simulink model "Engine"  (R2018a)
settings: Solver=VariableStepAuto  StartTime=0.0  StopTime=0  RelTol=1e-3
settings Model: Creator=josefl  LastModifiedBy=josefl

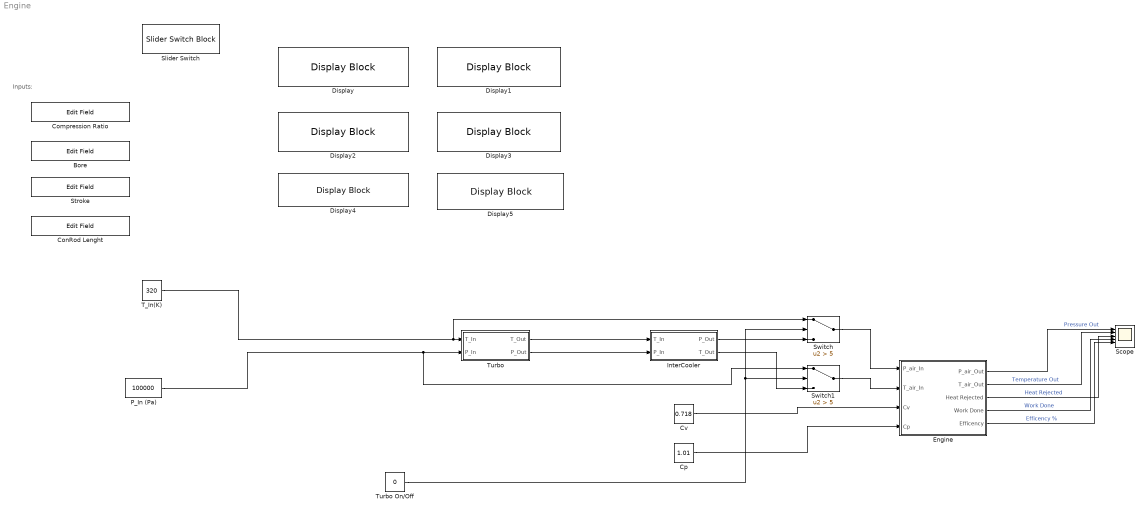
== system Engine ==
  note: Inputs:
  Bore : EditField  WebBlockId=61  LabelPosition=Hide  Alignment=Center
  "Compression Ratio " : EditField  WebBlockId=60  LabelPosition=Hide  Alignment=Center
  ConRod Lenght : EditField  WebBlockId=93  LabelPosition=Hide  Alignment=Center
  "Cp " : Constant  Value=1.01
  Cv : Constant  Value=0.718
  Display : DisplayBlock  WebBlockId=84
  Display1 : DisplayBlock  WebBlockId=85
  Display2 : DisplayBlock  WebBlockId=86
  Display3 : DisplayBlock  WebBlockId=87
  Display4 : DisplayBlock  WebBlockId=88
  Display5 : DisplayBlock  WebBlockId=89  LabelPosition=Hide
  "Engine " : Subsystem
  InterCooler : Subsystem
  "P_In (Pa) " : Constant  Value=100000
  Scope : Scope  NumInputPorts=5
  Slider Switch : SliderSwitchBlock  WebBlockId=64
      settings: Values={{'Off', 'On'}, [0 6]}
  "Stroke " : EditField  WebBlockId=62  LabelPosition=Hide  Alignment=Center
  Switch : Switch  Criteria=u2 > Threshold  Threshold=5
  Switch1 : Switch  Criteria=u2 > Threshold  Threshold=5
  "T_In(K) " : Constant  Value=320
  "Turbo " : Subsystem
  "Turbo On/Off " : Constant  Value=0
  wires:
  "Engine "/1("P_air_Out ") -> Scope/1  "Pressure Out"
  "Engine "/2("T_air_Out ") -> Scope/2  "Temperature Out"
  Cv/1 -> "Engine "/3(Cv)
  "Cp "/1 -> "Engine "/4("Cp ")
  "Engine "/3("Heat Rejected ") -> Scope/3  "Heat Rejected"
  "Engine "/4(Work Done) -> Scope/4  "Work Done"
  "Engine "/5(Efficency) -> Scope/5  "Efficency %"
  "P_In (Pa) "/1 -> Switch1/1, "Turbo "/2(P_In)
  "T_In(K) "/1 -> Switch/1, "Turbo "/1(T_In)
  "Turbo "/1(T_Out) -> InterCooler/1(T_In)
  "Turbo "/2(P_Out) -> InterCooler/2(P_In)
  InterCooler/1(P_Out) -> Switch/3
  Switch1/1 -> "Engine "/2("T_air_In ")
  Switch/1 -> "Engine "/1("P_air_In ")
  "Turbo On/Off "/1 -> Switch/2, Switch1/2
  InterCooler/2(T_Out) -> Switch1/3

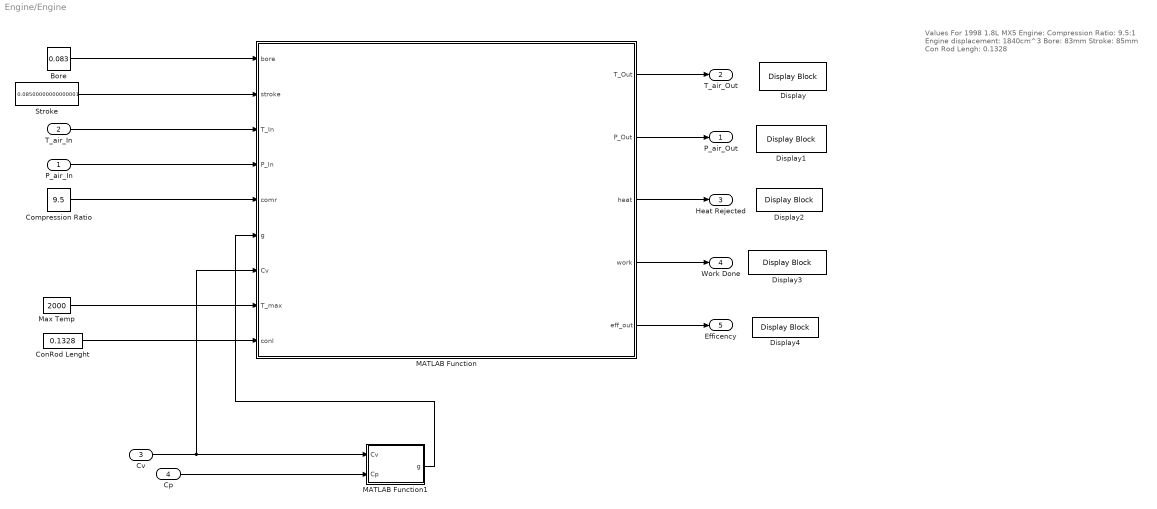
== system Engine/Engine  ==
  note: Values For 1998 1.8L MX5 Engine:
      | Compression Ratio: 9.5:1
      | Engine displacement: 1840cm^3
      | Bore: 83mm
      | Stroke: 85mm
      | Con Rod Lengh: 0.1328
  "P_air_In " : Inport
  "T_air_In " : Inport  Port=2
  Cv : Inport  Port=3
  "Cp " : Inport  Port=4
  "Bore " : Constant  Value=0.083
  "Compression Ratio " : Constant  Value=9.5
  ConRod Lenght : Constant  Value=0.1328
  Display : DisplayBlock  WebBlockId=50  LabelPosition=Hide
  Display1 : DisplayBlock  WebBlockId=51  LabelPosition=Hide
  Display2 : DisplayBlock  WebBlockId=55  LabelPosition=Hide
  Display3 : DisplayBlock  WebBlockId=56  LabelPosition=Hide
  Display4 : DisplayBlock  WebBlockId=57  LabelPosition=Hide
  MATLAB Function : MATLAB Function  TreatAsAtomicUnit=on
  MATLAB Function1 : MATLAB Function  TreatAsAtomicUnit=on
  "Max Temp " : Constant  Value=2000
  "Stroke " : Constant  Value=0.08500000000000001
  "P_air_Out " : Outport
  "T_air_Out " : Outport  Port=2
  "Heat Rejected " : Outport  Port=3
  Work Done : Outport  Port=4
  Efficency : Outport  Port=5
  wires:
  "Compression Ratio "/1 -> MATLAB Function/5(comr)
  "Bore "/1 -> MATLAB Function/1(bore)
  "Stroke "/1 -> MATLAB Function/2(stroke)
  "P_air_In "/1 -> MATLAB Function/4(P_In)
  "T_air_In "/1 -> MATLAB Function/3(T_In)
  MATLAB Function/2(P_Out) -> "P_air_Out "/1
  MATLAB Function/1(T_Out) -> "T_air_Out "/1
  Cv/1 -> MATLAB Function/7(Cv), MATLAB Function1/1(Cv)
  "Max Temp "/1 -> MATLAB Function/8(T_max)
  ConRod Lenght/1 -> MATLAB Function/9(conl)
  "Cp "/1 -> MATLAB Function1/2(Cp)
  MATLAB Function/3(heat) -> "Heat Rejected "/1
  MATLAB Function/4(work) -> Work Done/1
  MATLAB Function/5(eff_out) -> Efficency/1
  MATLAB Function1/1(g) -> MATLAB Function/6(g)

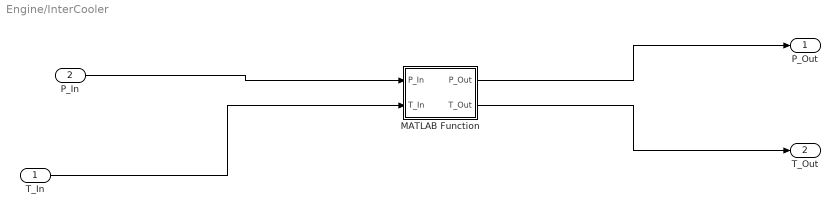
== system Engine/InterCooler ==
  T_In : Inport
  P_In : Inport  Port=2
  MATLAB Function : MATLAB Function  TreatAsAtomicUnit=on
  P_Out : Outport
  T_Out : Outport  Port=2
  wires:
  MATLAB Function/1(P_Out) -> P_Out/1
  T_In/1 -> MATLAB Function/2(T_In)
  MATLAB Function/2(T_Out) -> T_Out/1
  P_In/1 -> MATLAB Function/1(P_In)

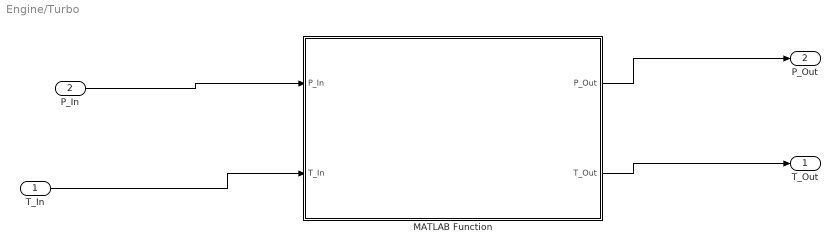
== system Engine/Turbo  ==
  T_In : Inport
  P_In : Inport  Port=2
  MATLAB Function : MATLAB Function  TreatAsAtomicUnit=on
  T_Out : Outport
  P_Out : Outport  Port=2
  wires:
  MATLAB Function/1(P_Out) -> P_Out/1
  T_In/1 -> MATLAB Function/2(T_In)
  MATLAB Function/2(T_Out) -> T_Out/1
  P_In/1 -> MATLAB Function/1(P_In)

== matlab function Engine/Engine /MATLAB Function1 ==
  data: Cv input; g output; Cp input
function g = fcn(Cv,Cp)
r1 = 1:1:10;
g1 = 1.5;
g2 = 1.4;
g3 = 1.3;
g = Cp/Cv;
e1 = (1-(1./(r1)).^(g1-1))*100;
e2 = (1-(1./(r1)).^(g2-1))*100;
e3 = (1-(1./(r1)).^(g3-1))*100;
e = (1-(1./(r1)).^(g-1))*100;

figure(2);
hold on 
plot(r1,e1,'color','b');
plot(r1,e2,'color','g');
plot(r1,e3,'color','r');
plot(r1,e,'color','black');
xlabel('Compression Ratio');
ylabel('Efficiency');
title('Theoretical Otto Cycle Efficency');

== matlab function Engine/Engine /MATLAB Function ==
  data: bore input; T_Out output; stroke input; T_In input; P_In input; comr input; P_Out output; g input; Cv input; T_max input; conl input; heat output; work output; eff_out output
function [T_Out,P_Out,heat,work,eff_out] = fcn(bore,stroke,T_In,P_In,comr,g,Cv,T_max,conl)

v_swept = (pi/4)*bore^2*stroke;
v_clearance = v_swept/(comr-1);

%State 1
p1 = P_In;
v1 = v_swept + v_clearance;
t1 = T_In;

%State 2 
v2 = v_clearance;
p2 = (p1*v1)/v2;
t2=t1*comr^(g-1);

%State 3 
v3 = v_clearance;
t3 = 2300;
p3 = (p2*t3)/t2;

%state 4 
v4 = v1;
p4 = p3/((comr)^g);
t4 = t3/(comr)^(g-1);

%overview Calcs
heat =Cv*(t4-t1);
h1 = (t3-t2)/Cv;
work =h1-heat;
eff = 1-(1/(comr)^(g-1));


%assigning output states 
T_Out = t4;
P_Out = p4;
eff_out = eff*100;

figure(1);
hold on
plot(v1,p1,'*','color','r')
plot(v2,p2,'*','color','g')
plot(v3,p3,'*','color','b')
plot(v4,p4,'*','color','y')
xlabel('Volume in m^3')
ylabel('Pressure in Pa')
title('Theoretical Otto Cycle PV diagram');
grid on

== matlab function Engine/Turbo /MATLAB Function ==
  data: P_In input; T_In input; P_Out output; T_Out output
function [P_Out,T_Out]= fcn(P_In,T_In)

P_Out = P_In;
T_Out = T_In;

== matlab function Engine/InterCooler/MATLAB Function ==
  data: P_In input; T_In input; P_Out output; T_Out output
function [P_Out,T_Out]= fcn(P_In,T_In)

P_Out = P_In/2;
T_Out = T_In/2;
